simulink model "extra"  (R2017a)
settings: Solver=VariableStepAuto  StartTime=0.0  StopTime=10.0  RelTol=1e-3
libraries: hdlsllib x8, simulink x4
settings Model: Creator=wachala.j  LastModifiedBy=wachala.j

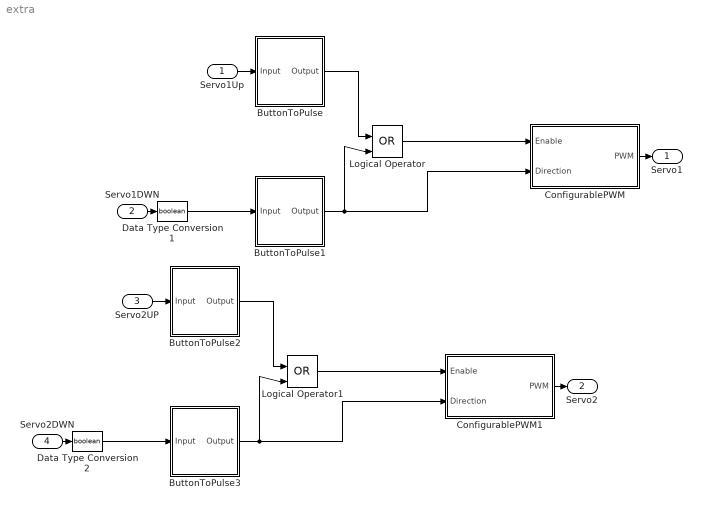
== system extra ==
  Servo1Up : Inport
  Servo1DWN : Inport  Port=2
  Servo2UP : Inport  Port=3
  Servo2DWN : Inport  Port=4
  ButtonToPulse : Subsystem
  ButtonToPulse1 : Subsystem
  ButtonToPulse2 : Subsystem
  ButtonToPulse3 : Subsystem
  ConfigurablePWM : Subsystem
  ConfigurablePWM1 : Subsystem
  Data Type Conversion1 : DataTypeConversion  OutDataTypeStr=boolean
  Data Type Conversion2 : DataTypeConversion  OutDataTypeStr=boolean
  Logical Operator : Logic  Operator=OR  IconShape=distinctive  AllPortsSameDT=off  OutDataTypeStr=boolean
  Logical Operator1 : Logic  Operator=OR  IconShape=distinctive  AllPortsSameDT=off  OutDataTypeStr=boolean
  Servo1 : Outport
  Servo2 : Outport  Port=2
  wires:
  Logical Operator/1 -> ConfigurablePWM/1(Enable)
  ButtonToPulse1/1(Output) -> Logical Operator/2, ConfigurablePWM/2(Direction)
  Servo1Up/1 -> ButtonToPulse/1(Input)
  Data Type Conversion1/1 -> ButtonToPulse1/1(Input)
  ConfigurablePWM/1(PWM) -> Servo1/1
  ButtonToPulse/1(Output) -> Logical Operator/1
  Servo1DWN/1 -> Data Type Conversion1/1
  Logical Operator1/1 -> ConfigurablePWM1/1(Enable)
  ButtonToPulse3/1(Output) -> Logical Operator1/2, ConfigurablePWM1/2(Direction)
  Servo2UP/1 -> ButtonToPulse2/1(Input)
  Data Type Conversion2/1 -> ButtonToPulse3/1(Input)
  ConfigurablePWM1/1(PWM) -> Servo2/1
  ButtonToPulse2/1(Output) -> Logical Operator1/1
  Servo2DWN/1 -> Data Type Conversion2/1

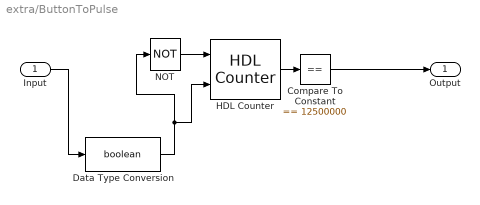
== system extra/ButtonToPulse ==
  Input : Inport
  Compare To Constant : simulink/Logic and Bit Operations/Compare To Constant  relop===  const=12500000  OutDataTypeStr=boolean
  Data Type Conversion : DataTypeConversion  OutDataTypeStr=boolean
  HDL Counter : hdlsllib/HDL Operations/HDL Counter  CountType=Count limited  CountInit=0  CountStep=1  CountMax=50000000  CountFromType=Initial value  CountFrom=0  CountResetPort=on  CountLoadPort=off  CountEnbPort=on  CountDirPort=off  CountDataType=Unsigned  CountWordLen=32  CountFracLen=0  CountSampTime=1
      settings: SourceProductName=HDL Coder  SourceProductBaseCode=HD
  NOT : Logic  Operator=NOT  IconShape=distinctive  AllPortsSameDT=off  OutDataTypeStr=boolean
  Output : Outport
  wires:
  NOT/1 -> HDL Counter/1
  Data Type Conversion/1 -> HDL Counter/2, NOT/1
  HDL Counter/1 -> Compare To Constant/1
  Input/1 -> Data Type Conversion/1
  Compare To Constant/1 -> Output/1

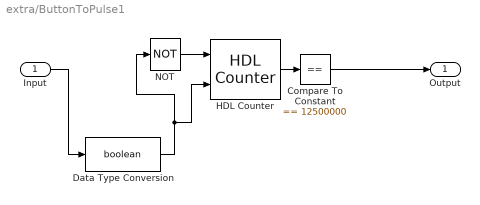
== system extra/ButtonToPulse1 ==
  Input : Inport
  Compare To Constant : simulink/Logic and Bit Operations/Compare To Constant  relop===  const=12500000  OutDataTypeStr=boolean
  Data Type Conversion : DataTypeConversion  OutDataTypeStr=boolean
  HDL Counter : hdlsllib/HDL Operations/HDL Counter  CountType=Count limited  CountInit=0  CountStep=1  CountMax=50000000  CountFromType=Initial value  CountFrom=0  CountResetPort=on  CountLoadPort=off  CountEnbPort=on  CountDirPort=off  CountDataType=Unsigned  CountWordLen=32  CountFracLen=0  CountSampTime=1
      settings: SourceProductName=HDL Coder  SourceProductBaseCode=HD
  NOT : Logic  Operator=NOT  IconShape=distinctive  AllPortsSameDT=off  OutDataTypeStr=boolean
  Output : Outport
  wires:
  NOT/1 -> HDL Counter/1
  Data Type Conversion/1 -> HDL Counter/2, NOT/1
  HDL Counter/1 -> Compare To Constant/1
  Input/1 -> Data Type Conversion/1
  Compare To Constant/1 -> Output/1

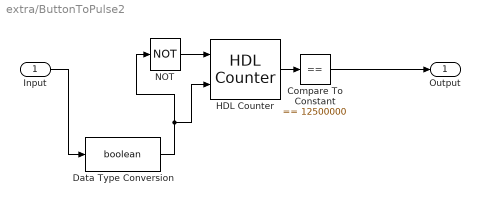
== system extra/ButtonToPulse2 ==
  Input : Inport
  Compare To Constant : simulink/Logic and Bit Operations/Compare To Constant  relop===  const=12500000  OutDataTypeStr=boolean
  Data Type Conversion : DataTypeConversion  OutDataTypeStr=boolean
  HDL Counter : hdlsllib/HDL Operations/HDL Counter  CountType=Count limited  CountInit=0  CountStep=1  CountMax=50000000  CountFromType=Initial value  CountFrom=0  CountResetPort=on  CountLoadPort=off  CountEnbPort=on  CountDirPort=off  CountDataType=Unsigned  CountWordLen=32  CountFracLen=0  CountSampTime=1
      settings: SourceProductName=HDL Coder  SourceProductBaseCode=HD
  NOT : Logic  Operator=NOT  IconShape=distinctive  AllPortsSameDT=off  OutDataTypeStr=boolean
  Output : Outport
  wires:
  NOT/1 -> HDL Counter/1
  Data Type Conversion/1 -> HDL Counter/2, NOT/1
  HDL Counter/1 -> Compare To Constant/1
  Input/1 -> Data Type Conversion/1
  Compare To Constant/1 -> Output/1

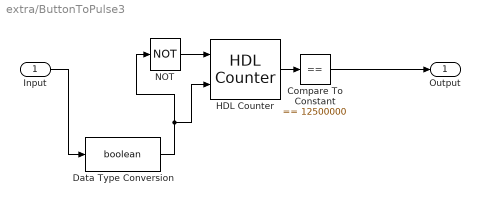
== system extra/ButtonToPulse3 ==
  Input : Inport
  Compare To Constant : simulink/Logic and Bit Operations/Compare To Constant  relop===  const=12500000  OutDataTypeStr=boolean
  Data Type Conversion : DataTypeConversion  OutDataTypeStr=boolean
  HDL Counter : hdlsllib/HDL Operations/HDL Counter  CountType=Count limited  CountInit=0  CountStep=1  CountMax=50000000  CountFromType=Initial value  CountFrom=0  CountResetPort=on  CountLoadPort=off  CountEnbPort=on  CountDirPort=off  CountDataType=Unsigned  CountWordLen=32  CountFracLen=0  CountSampTime=1
      settings: SourceProductName=HDL Coder  SourceProductBaseCode=HD
  NOT : Logic  Operator=NOT  IconShape=distinctive  AllPortsSameDT=off  OutDataTypeStr=boolean
  Output : Outport
  wires:
  NOT/1 -> HDL Counter/1
  Data Type Conversion/1 -> HDL Counter/2, NOT/1
  HDL Counter/1 -> Compare To Constant/1
  Input/1 -> Data Type Conversion/1
  Compare To Constant/1 -> Output/1

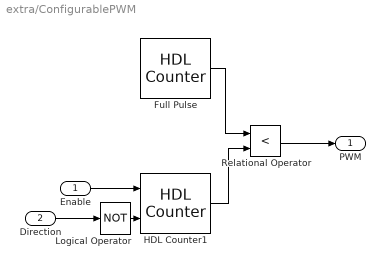
== system extra/ConfigurablePWM ==
  Enable : Inport  OutDataTypeStr=boolean
  Direction : Inport  Port=2  OutDataTypeStr=boolean
  Full Pulse : hdlsllib/HDL Operations/HDL Counter  CountType=Count limited  CountInit=0  CountStep=1  CountMax=1000000  CountFromType=Initial value  CountFrom=0  CountResetPort=off  CountLoadPort=off  CountEnbPort=off  CountDirPort=off  CountDataType=Unsigned  CountWordLen=32  CountFracLen=0  CountSampTime=1
      settings: SourceProductName=HDL Coder  SourceProductBaseCode=HD
  HDL Counter1 : hdlsllib/HDL Operations/HDL Counter  CountType=Count limited  CountInit=30  CountStep=6  CountMax=120  CountFromType=Initial value  CountFrom=30  CountResetPort=off  CountLoadPort=off  CountEnbPort=on  CountDirPort=on  CountDataType=Unsigned  CountWordLen=8  CountFracLen=0  CountSampTime=1
      settings: SourceProductName=HDL Coder  SourceProductBaseCode=HD
  Logical Operator : Logic  Operator=NOT  IconShape=distinctive  AllPortsSameDT=off  OutDataTypeStr=boolean
  Relational Operator : RelationalOperator  Operator=<  OutDataTypeStr=boolean  RndMeth=Simplest
  PWM : Outport
  wires:
  Relational Operator/1 -> PWM/1
  HDL Counter1/1 -> Relational Operator/2
  Full Pulse/1 -> Relational Operator/1
  Enable/1 -> HDL Counter1/1
  Direction/1 -> Logical Operator/1
  Logical Operator/1 -> HDL Counter1/2

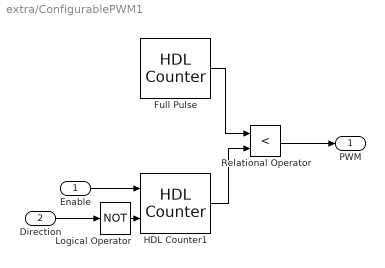
== system extra/ConfigurablePWM1 ==
  Enable : Inport  OutDataTypeStr=boolean
  Direction : Inport  Port=2  OutDataTypeStr=boolean
  Full Pulse : hdlsllib/HDL Operations/HDL Counter  CountType=Count limited  CountInit=0  CountStep=1  CountMax=1000000  CountFromType=Initial value  CountFrom=0  CountResetPort=off  CountLoadPort=off  CountEnbPort=off  CountDirPort=off  CountDataType=Unsigned  CountWordLen=32  CountFracLen=0  CountSampTime=1
      settings: SourceProductName=HDL Coder  SourceProductBaseCode=HD
  HDL Counter1 : hdlsllib/HDL Operations/HDL Counter  CountType=Count limited  CountInit=30  CountStep=6  CountMax=120  CountFromType=Initial value  CountFrom=30  CountResetPort=off  CountLoadPort=off  CountEnbPort=on  CountDirPort=on  CountDataType=Unsigned  CountWordLen=8  CountFracLen=0  CountSampTime=1
      settings: SourceProductName=HDL Coder  SourceProductBaseCode=HD
  Logical Operator : Logic  Operator=NOT  IconShape=distinctive  AllPortsSameDT=off  OutDataTypeStr=boolean
  Relational Operator : RelationalOperator  Operator=<  OutDataTypeStr=boolean  RndMeth=Simplest
  PWM : Outport
  wires:
  Relational Operator/1 -> PWM/1
  HDL Counter1/1 -> Relational Operator/2
  Full Pulse/1 -> Relational Operator/1
  Enable/1 -> HDL Counter1/1
  Direction/1 -> Logical Operator/1
  Logical Operator/1 -> HDL Counter1/2
